simulink model "BitwiseNOR_int8"  (R2017b)
settings: Solver=FixedStepDiscrete  StartTime=0.0  StopTime=10.0  FixedStep=0.200000  RelTol=1e-3  EnableMultiTasking=on
model workspace (MAT data in the model file):
  already_pp = 0
  input_struct.time = [0; 0.2; 0.4; 0.6; 0.8; 1; 1.2; 1.4; 1.6; 1.8; 2; 2.2; 2.4; 2.6; 2.8; 3; 3.2; 3.4; 3.6; 3.8; 4; 4.2; 4.4; 4.6; 4.8; 5; 5.2; 5.4; 5.6; 5.8; 6; 6.2; 6.4; 6.6; 6.8; 7; 7.2; 7.4; 7.6; 7.8; 8; 8.2; 8.4; 8.6; 8.8; 9; 9.2; 9.4; 9.6; 9.8; 10; 10.2; 10.4; 10.6; 10.8; 11; 11.2; 11.4; 11.6; 11.8; 12; 12.2; 12.4; 12.6; 12.8; 13; 13.2; 13.4; 13.6; 13.8; 14; 14.2; 14.4; 14.6; 14.8; 15; 15.2; 15.4; 15.6; 15.8; 16; 16.2; 16.4; 16.6; 16.8; 17; 17.2; 17.4; 17.6; 17.8; 18; 18.2; 18.4; 18.6; 18.8; 19; 19.2; 19.4; 19.6; 19.8]
  input_struct.signals(1).name = 'In1'
  input_struct.signals(1).values = [77; -10; 16; 25; -52; -74; -50; -54; -50; -59; 58; -7; -84; -89; 30; -77; 0; 24; -55; 93; 50; -22; -41; 80; -23; -98; -74; 27; 10; -50; -21; -65; 53; 59; -4; -83; 24; 95; 0; -5; 100; 44; -6; -97; 3; 40; -85; -84; 25; -17; -16; 8; -85; 14; 67; -41; 29; -73; 69; 65; 51; 84; -10; 41; 35; -19; 82; 73; -53; 13; 0; 90; -97; -38; 94; 70; -81; -92; 82; 11; 69; -37; 4; -61; -98; 90; 7; -80; -10; 50; 6; 86; -21; -68; 70; -68; 71; 69; -3; 55]
  input_struct.signals(1).dimensions = 1
  input_struct.signals(2).name = 'In2'
  input_struct.signals(2).values = [69; -20; 12; 3; -42; 85; -19; 82; -3; -18; 40; 68; -62; 74; 23; -12; 31; -77; 43; -80; 14; 48; 84; 76; -26; 42; -24; -11; -54; 17; -98; -18; -23; -72; 48; -35; -24; 98; 25; -19; -54; 94; -71; -20; 6; -80; 16; -79; 19; -4; 64; 15; -58; -14; -14; 75; 50; -21; -67; 8; -96; -76; 27; -3; 99; 32; 95; 77; 41; -84; -12; -100; 36; 55; 83; -29; 9; 31; -65; 97; -100; -61; -6; 11; -49; 99; -11; -89; 39; -53; -40; -49; -83; 14; -47; -94; 28; 20; -62; 38]
  input_struct.signals(2).dimensions = 1
  input_struct.signals(3).name = 'In3'
  input_struct.signals(3).values = [-38; -15; -24; 25; 57; 19; 30; 18; -69; -92; -73; -44; 52; -17; -71; 47; 34; 27; 9; -50; -86; -23; 91; -96; 18; 77; 16; 43; 44; -24; -69; -69; -8; -93; 46; 51; -10; -43; -72; -1; -27; 56; -72; 50; 24; 82; 44; -77; 75; -87; -100; -39; -21; -43; 30; -48; 98; 35; 34; 58; -87; -52; 2; 74; 100; 22; -96; 82; 58; 2; 51; 22; -16; -51; -59; -35; -29; -18; 3; 82; -77; -64; -6; -38; 87; 76; 98; -61; 64; 23; -53; 59; -13; -74; 14; -75; -57; -6; -2; -62]
  input_struct.signals(3).dimensions = 1
  input_struct.signals(4).name = 'In4'
  input_struct.signals(4).values = [-76  -33  -27; 35  -64  85; 99  -13  40; 32  52  99; -55  84  94; 66  0  -82; -26  -25  -26; 40  55  6; 29  -62  -84; -95  -5  41; -41  16  -31; 82  72  -78; 32  34  89; -40  -62  -59; 16  87  -99; -26  20  74; -67  31  36; -92  -25  -66; 97  -35  -65; 17  -94  80; 24  -12  -84; -44  65  -86; 81  31  -96; -12  99  15; -52  20  -35; -92  4  5; -76  -86  -20; -1  33  26; 40  -18  26; -36  -48  -32; -98  53  92; 30  77  -33; -62  10  34; 4  -10  -95; 86  87  73; -7  -84  -33; 74  -27  84; -16  -94  -51; 78  -91  -85; -26  28  -44; -74  2  -40; -14  12  25; -22  -44  16; 97  36  39; 96  25  -72; -39  42  -31; 87  23  25; 60  -10  72; 88  46  -6; 24  97  38; -27  7  -82; -18  56  -89; 44  99  65; 27  27  -82; 15  -46  -59; 63  21  59; -71  27  37; -47  83  -6; -25  23  80; -80  89  -18; 48  -49  32; -35  -61  92; 19  -11  -40; 79  76  45; -43  -30  51; 49  -79  -63; -5  53  14; -17  80  -88; 66  -63  37; 5  35  34; -5  3  -74; 73  73  79; -74  -41  -66; -75  -40  9; -74  -56  -94; 31  -72  63; 96  92  19; 18  36  -19; -17  61  29; -99  7  -27; 80  65  100; 96  -48  41; 99  39  -61; 85  71  66; -64  -83  -40; 12  94  5; 0  40  25; 73  -85  -100; -26  89  55; 81  93  -58; 23  -22  -60; 55  15  59; 47  64  -46; 95  -85  66; 59  73  100; -8  -64  -21; 53  67  80; 95  69  6; -49  2  -84; 84  4  -16]
  input_struct.signals(4).dimensions = 3
  input_struct.signals(5).name = 'In5'
  input_struct.signals(5).values = [-97  -26  -67; 81  8  -64; -25  -50  90; -98  44  27; 0  -36  9; -11  -93  29; 71  63  99; 0  -91  63; -78  -41  83; 59  -39  12; 87  7  -38; 72  -76  -11; -69  59  -47; -84  1  -72; 26  -55  54; -81  67  22; -94  -78  -57; -35  100  -6; 29  52  59; 17  4  17; 35  -5  83; 59  -46  51; -24  93  62; -85  -36  46; -13  -9  69; 57  7  23; -39  57  23; 47  -18  -99; -80  82  13; -66  -76  71; 85  75  -10; 58  30  -33; 56  -14  -83; 76  -73  79; 82  -97  -11; 87  -27  79; -19  -97  5; -42  -6  -9; 54  -74  -98; 89  69  -47; -44  92  60; -26  -61  -59; -46  48  29; -5  -89  39; 93  3  -81; -80  -77  48; 8  29  96; -39  -68  52; -70  -88  -59; -16  12  -65; -35  -71  83; 11  -26  -46; -63  -60  -62; -57  -100  -13; 13  62  83; 82  81  -62; 40  -12  42; 77  -27  53; 49  -27  -46; -11  -43  -41; -77  67  93; 88  96  -58; 19  -57  -24; -34  33  34; -42  -12  -25; 1  -18  37; 69  70  96; 90  0  34; 70  -54  40; 9  43  -51; 4  -14  75; 5  -17  56; 25  87  -72; -44  -71  -50; 4  -97  11; -34  -15  2; -45  90  96; -26  46  56; 98  -38  -52; 51  -69  -83; -11  98  61; 70  71  41; 0  35  86; 10  -46  -20; 49  81  -49; -46  -47  48; -23  71  -19; 51  -16  8; -1  -83  -69; 33  88  94; 81  65  13; -33  87  -74; -41  28  6; 24  98  -53; -64  26  72; -58  -14  84; 62  -45  17; -79  66  -32; 36  86  99; -61  91  36]
  input_struct.signals(5).dimensions = 3
  input_struct.signals(6).name = 'In6'
  input_struct.signals(6).values = [-65  -71  56; -53  24  36; 48  87  -68; 11  28  -50; -93  84  96; 11  48  55; 96  -24  70; 42  -28  -26; 94  86  36; 80  -19  -14; 16  -97  31; 43  -83  36; 69  41  90; 38  80  1; -68  66  -11; -72  -3  -81; -31  -45  -10; 63  -7  64; -100  41  -18; -53  53  20; -94  99  -83; 36  44  -77; 71  -9  99; 54  3  31; 15  -29  27; -46  -3  74; 84  42  -45; 68  64  33; 86  48  -85; 78  90  -89; 53  -30  74; 22  34  78; 50  78  97; -41  38  80; 44  53  -75; 81  11  -69; -92  -87  63; -32  15  4; -53  -60  59; -86  4  22; -10  91  54; -86  -77  89; 81  94  33; -10  72  47; 6  -89  -50; 95  62  -81; 60  -45  55; 5  -97  42; -36  -29  41; 68  27  -55; -88  -28  84; -59  3  -6; -43  100  13; 47  44  27; 14  75  38; 25  -15  -86; -49  -7  96; -66  -74  -88; -52  -82  -44; -82  -4  -8; 71  86  64; 76  -11  -65; 38  -38  -95; -53  -51  89; 23  88  -22; -38  -32  -74; -10  74  65; -68  86  72; -55  -33  54; -92  -46  78; -41  5  40; -5  20  30; -31  13  -13; 66  -76  -1; -72  13  -5; -83  -5  17; 82  -46  44; 81  97  5; -53  -58  -40; 2  -50  -20; 10  91  -32; 28  49  -47; 15  2  -12; 6  -9  -80; 84  -38  -71; -97  43  72; -59  82  13; 17  -11  -80; 48  55  26; 5  14  -4; 92  -79  71; 98  -19  85; 60  -33  -35; 46  -48  91; -69  -7  47; 70  15  -82; -90  71  -27; 29  -95  -15; -12  47  98; -98  -54  56]
  input_struct.signals(6).dimensions = 3
settings Model: Creator=hbourbou  LastModifiedBy=hbourbou
settings OptimizationCC: LifeSpan=inf
settings DebuggingCC: AlgebraicLoopMsg=error  ArtificialAlgebraicLoopMsg=error  SFExecutionAtInitializationDiag=none
settings HardwareCC: ProdBitPerSizeT=32  ProdBitPerPtrDiffT=32  ProdWordSize=32  ProdHWDeviceType=Specified
settings CodeAppCC: StateflowObjectComments=on

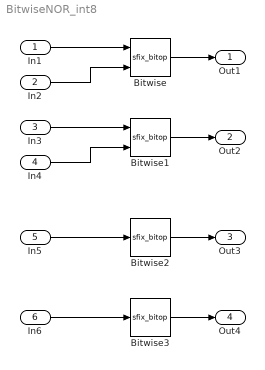
== system BitwiseNOR_int8 ==
  In1 : Inport  OutDataTypeStr=int8  PortDimensions=1
  In2 : Inport  Port=2  OutDataTypeStr=int8  PortDimensions=1
  In3 : Inport  Port=3  OutDataTypeStr=int8  PortDimensions=1
  In4 : Inport  Port=4  OutDataTypeStr=int8  PortDimensions=3
  In5 : Inport  Port=5  OutDataTypeStr=int8  PortDimensions=3
  In6 : Inport  Port=6  OutDataTypeStr=int8  PortDimensions=3
  Bitwise : S-Function  FunctionName=sfix_bitop  Parameters=UseBitMask,NumInputPorts,BitMask,BitMaskRealWorld,logicop  SFunctionDeploymentMode=off  EnableBusSupport=off  mask(Bitwise Operator){logicop=NOR, UseBitMask=off, NumInputPorts=2, BitMask=bin2dec('11011001'), BitMaskRealWorld=Stored Integer}
      mask prompts: logicop "Simulink:masks:Operator_MP"; UseBitMask "Simulink:masks:UseBitMask_MP"; NumInputPorts "Simulink:masks:NumberOfInputPorts_MP"; BitMask "Simulink:masks:BitMask_MP"; BitMaskRealWorld "Simulink:masks:TreatMaskAs_MP"
      mask help: Simulink:masks:BitwiseOperator_MD
      mask init:
      | str = '';
      | if UseBitMask
      |   [m,n] = size(BitMask);
      |   if ischar(BitMask)
      |     len = m;
      |     n = 1;
      |   else
      |     len = m * n;
      |   end
      |   internalBitMask = zeros(m,n);
      |   if isnumeric(BitMask)
      |     if ~isreal(BitMask)
      |       error(DAStudio.message('Simulink:blocks:BitMaskNotComplex'));
      |     end
      |     for i=1:len,
      |       internalBitMask(i) = BitMask(i);
      |     end
      |   elseif ischar(BitMask)
      |     for i=1:m,
      |       internalBitMask(i) = hex2dec(BitMask(i,:));
      |     end
      |   elseif iscell(BitMask)
      |     for i=1:len,
      |       if isnumeric( BitMask{i} )
      |         internalBitMask(i) = BitMask{i};
      |       elseif ischar( BitMask{i} )
      |         internalBitMask(i) = hex2dec(BitMask{i});
      |       else
      |         errordlg(['Data type is not supported at cell item ', num2str(i) ]);
      |       end
      |     end
      |   end
      |   BitMask = internalBitMask;
      |   for i=1:len
      |     if BitMask(i) > (2^52)-1
      |       error(DAStudio.message('Simulink:blocks:BitMaskWordLengthTooLarge')); 
      |     end
      |   end 
      |   if len == 1
      |      if BitMaskRealWorld == 1 || BitMask(1) < 0
      |        str=num2str(BitMask(1));
      |      else
      |        str=['0x',dec2hex(floor(BitMask(1)))];
      |      end
      |   else
      |      str='Masks';
      |   end
      | else
      |   BitMask = 0;
      |   str='';
      | end
      mask TypeOptions logicop: Simulink:masks:AND | Simulink:masks:OR | Simulink:masks:NAND | Simulink:masks:NOR | Simulink:masks:XOR | Simulink:masks:NOT
      mask Callback logicop: fixptdialog(gcbh)
      mask Callback UseBitMask: fixptdialog(gcbh)
      mask TypeOptions BitMaskRealWorld: Simulink:masks:RealWorldValue | Simulink:masks:StoredInteger
      mask Display: fprintf(['Bitwise\n',logicop,'\n',str])
  Bitwise1 : S-Function  FunctionName=sfix_bitop  Parameters=UseBitMask,NumInputPorts,BitMask,BitMaskRealWorld,logicop  SFunctionDeploymentMode=off  EnableBusSupport=off  mask(Bitwise Operator){logicop=NOR, UseBitMask=off, NumInputPorts=2, BitMask=bin2dec('11011001'), BitMaskRealWorld=Stored Integer}
      mask prompts: logicop "Simulink:masks:Operator_MP"; UseBitMask "Simulink:masks:UseBitMask_MP"; NumInputPorts "Simulink:masks:NumberOfInputPorts_MP"; BitMask "Simulink:masks:BitMask_MP"; BitMaskRealWorld "Simulink:masks:TreatMaskAs_MP"
      mask help: Simulink:masks:BitwiseOperator_MD
      mask init: same as BitwiseNOR_int8/Bitwise
      mask TypeOptions logicop: Simulink:masks:AND | Simulink:masks:OR | Simulink:masks:NAND | Simulink:masks:NOR | Simulink:masks:XOR | Simulink:masks:NOT
      mask Callback logicop: fixptdialog(gcbh)
      mask Callback UseBitMask: fixptdialog(gcbh)
      mask TypeOptions BitMaskRealWorld: Simulink:masks:RealWorldValue | Simulink:masks:StoredInteger
      mask Display: fprintf(['Bitwise\n',logicop,'\n',str])
  Bitwise2 : S-Function  FunctionName=sfix_bitop  Parameters=UseBitMask,NumInputPorts,BitMask,BitMaskRealWorld,logicop  SFunctionDeploymentMode=off  EnableBusSupport=off  mask(Bitwise Operator){logicop=NOR, UseBitMask=on, NumInputPorts=1, BitMask=bin2dec('11011001'), BitMaskRealWorld=Stored Integer}
      mask prompts: logicop "Simulink:masks:Operator_MP"; UseBitMask "Simulink:masks:UseBitMask_MP"; NumInputPorts "Simulink:masks:NumberOfInputPorts_MP"; BitMask "Simulink:masks:BitMask_MP"; BitMaskRealWorld "Simulink:masks:TreatMaskAs_MP"
      mask help: Simulink:masks:BitwiseOperator_MD
      mask init: same as BitwiseNOR_int8/Bitwise
      mask TypeOptions logicop: Simulink:masks:AND | Simulink:masks:OR | Simulink:masks:NAND | Simulink:masks:NOR | Simulink:masks:XOR | Simulink:masks:NOT
      mask Callback logicop: fixptdialog(gcbh)
      mask Callback UseBitMask: fixptdialog(gcbh)
      mask TypeOptions BitMaskRealWorld: Simulink:masks:RealWorldValue | Simulink:masks:StoredInteger
      mask Display: fprintf(['Bitwise\n',logicop,'\n',str])
  Bitwise3 : S-Function  FunctionName=sfix_bitop  Parameters=UseBitMask,NumInputPorts,BitMask,BitMaskRealWorld,logicop  SFunctionDeploymentMode=off  EnableBusSupport=off  mask(Bitwise Operator){logicop=NOR, UseBitMask=off, NumInputPorts=1, BitMask=bin2dec('11011001'), BitMaskRealWorld=Stored Integer}
      mask prompts: logicop "Simulink:masks:Operator_MP"; UseBitMask "Simulink:masks:UseBitMask_MP"; NumInputPorts "Simulink:masks:NumberOfInputPorts_MP"; BitMask "Simulink:masks:BitMask_MP"; BitMaskRealWorld "Simulink:masks:TreatMaskAs_MP"
      mask help: Simulink:masks:BitwiseOperator_MD
      mask init: same as BitwiseNOR_int8/Bitwise
      mask TypeOptions logicop: Simulink:masks:AND | Simulink:masks:OR | Simulink:masks:NAND | Simulink:masks:NOR | Simulink:masks:XOR | Simulink:masks:NOT
      mask Callback logicop: fixptdialog(gcbh)
      mask Callback UseBitMask: fixptdialog(gcbh)
      mask TypeOptions BitMaskRealWorld: Simulink:masks:RealWorldValue | Simulink:masks:StoredInteger
      mask Display: fprintf(['Bitwise\n',logicop,'\n',str])
  Out1 : Outport
  Out2 : Outport  Port=2
  Out3 : Outport  Port=3
  Out4 : Outport  Port=4
  wires:
  In1/1 -> Bitwise/1
  In2/1 -> Bitwise/2
  Bitwise/1 -> Out1/1
  Bitwise1/1 -> Out2/1
  In3/1 -> Bitwise1/1
  In4/1 -> Bitwise1/2
  In5/1 -> Bitwise2/1
  Bitwise2/1 -> Out3/1
  Bitwise3/1 -> Out4/1
  In6/1 -> Bitwise3/1
